simulink model "Therac_Mcode"  (Simulink 8.7)
settings: Solver=FixedStepDiscrete  StartTime=0.0  StopTime=10.0  FixedStep=1  RelTol=1e-3
undefined symbols (not defined in the file or in its folder): sldvsubsys
libraries: simulink x7, sldvlib x2
settings DebuggingCC: SolverPrmCheckMsg=warning  AllowSymbolicDim=off
settings ConfigComp: DVMaxProcessTime=3000  DVMaxTestCaseSteps=500  DVTestSuiteOptimization=CombinedObjectives (Nonlinear Extended)  DVDetectActiveLogic=on

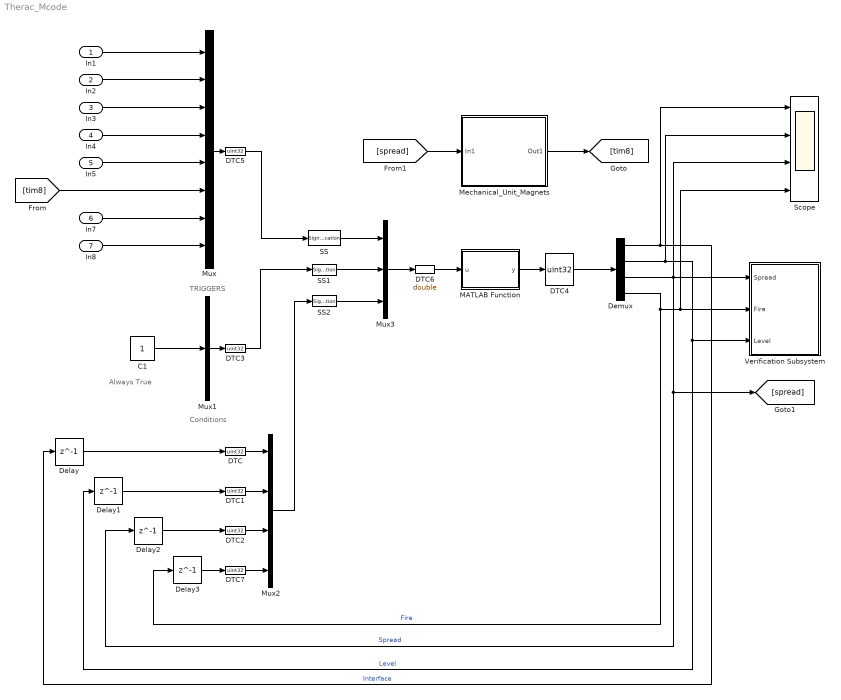
== system Therac_Mcode ==
  note: Always True
  note: Conditions
  note: TRIGGERS
  In1 : Inport  OutDataTypeStr=boolean
  In2 : Inport  Port=2  OutDataTypeStr=boolean
  In3 : Inport  Port=3  OutDataTypeStr=boolean
  In4 : Inport  Port=4  OutDataTypeStr=boolean
  In5 : Inport  Port=5  OutDataTypeStr=boolean
  In7 : Inport  Port=6  OutDataTypeStr=boolean
  In8 : Inport  Port=7  OutDataTypeStr=boolean
  C1 : Constant
  DTC{,1..5,7} (7 alike) : DataTypeConversion  OutDataTypeStr=uint32
  DTC6 : DataTypeConversion  OutDataTypeStr=double
  Delay{,1..3} (4 alike) : Delay  DelayLength=1  InitialCondition=1
  Demux : Demux
  MATLAB Function : MATLAB Function  TreatAsAtomicUnit=on
  Mechanical_Unit_Magnets : Subsystem
  Mux : Mux  Inputs=8
  Mux1 : Mux  Inputs=1
  Mux2 : Mux
  Mux3 : Mux  Inputs=3
  SS : SignalSpecification  Dimensions=8
  SS1 : SignalSpecification  Dimensions=1
  SS2 : SignalSpecification  Dimensions=4
  Scope : Scope  NumInputPorts=4
  Verification Subsystem : Subsystem  Tag=VerificationSubsystem  DisableCoverage=on  LoadFcn=sldvsubsys('check')  TreatAsAtomicUnit=on  SimViewingDevice=on  mask(VerificationSubsystem){}
      mask init:
      | sldvsubsys('maskInit');
      settings: CopyFcn=sldvsubsys('copy');  OpenFcn=open_system(gcb,'force');
      settings: PreSaveFcn=|
      | set_param(gcb,'SimViewingDevice','on');
      | sldvsubsys('check');
      mask Help: helpview(fullfile(docroot,'toolbox','sldv','sldv.map'),'verificationsubsystem')
      mask Display: image(imread('sldvicon_versubsys.png','BackGroundColor',[1 1 1]),'center');
  wires:
  Demux/2 -> Scope/2, Verification Subsystem/3(Level), Delay1/1  "Level"
  Delay2/1 -> DTC2/1
  Mux1/1 -> DTC3/1
  Delay1/1 -> DTC1/1
  Mux/1 -> DTC5/1
  Delay/1 -> DTC/1
  Mux3/1 -> DTC6/1
  Mux2/1 -> SS2/1
  Demux/1 -> Scope/1, Delay/1  "Interface"
  In7/1 -> Mux/7
  In3/1 -> Mux/3
  In2/1 -> Mux/2
  In4/1 -> Mux/4
  In5/1 -> Mux/5
  [tim8] -> Mux/6
  In8/1 -> Mux/8
  MATLAB Function/1(y) -> DTC4/1
  Demux/3 -> Scope/3, Delay2/1, [spread], Verification Subsystem/1(Spread)  "Spread"
  SS/1 -> Mux3/1
  SS1/1 -> Mux3/2
  DTC4/1 -> Demux/1
  DTC/1 -> Mux2/1
  DTC1/1 -> Mux2/2
  DTC2/1 -> Mux2/3
  DTC3/1 -> SS1/1
  SS2/1 -> Mux3/3
  DTC5/1 -> SS/1
  DTC6/1 -> MATLAB Function/1(u)
  In1/1 -> Mux/1
  Delay3/1 -> DTC7/1
  DTC7/1 -> Mux2/4
  Demux/4 -> Delay3/1, Scope/4, Verification Subsystem/2(Fire)  "Fire"
  C1/1 -> Mux1/1
  Mechanical_Unit_Magnets/1(Out1) -> [tim8]
  [spread] -> Mechanical_Unit_Magnets/1(In1)

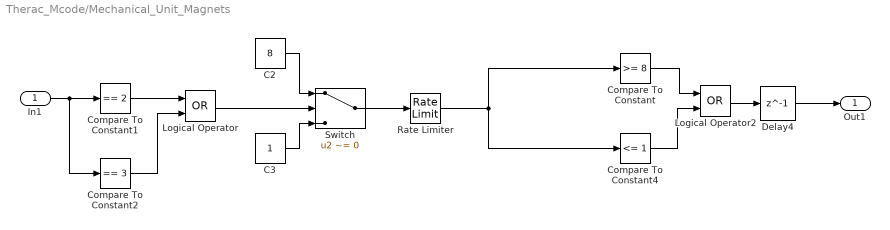
== system Therac_Mcode/Mechanical_Unit_Magnets ==
  In1 : Inport
  C2 : Constant  Value=8
  C3 : Constant
  Compare To Constant : simulink/Logic and Bit Operations/Compare To Constant  relop=>=  const=8  OutDataTypeStr=boolean
  Compare To Constant1 : simulink/Logic and Bit Operations/Compare To Constant  relop===  const=2  OutDataTypeStr=boolean
  Compare To Constant2 : simulink/Logic and Bit Operations/Compare To Constant  relop===  const=3  OutDataTypeStr=boolean
  Compare To Constant4 : simulink/Logic and Bit Operations/Compare To Constant  relop=<=  const=1  OutDataTypeStr=boolean
  Delay4 : Delay  DelayLength=1  InitialCondition=0
  Logical Operator : Logic  Operator=OR  AllPortsSameDT=off  OutDataTypeStr=boolean
  Logical Operator2 : Logic  Operator=OR  AllPortsSameDT=off  OutDataTypeStr=boolean
  Rate Limiter : RateLimiter  SampleTimeMode=inherited
  Switch : Switch  Criteria=u2 ~= 0
  Out1 : Outport
  wires:
  Switch/1 -> Rate Limiter/1
  C3/1 -> Switch/3
  Compare To Constant/1 -> Logical Operator2/1
  Logical Operator/1 -> Switch/2
  Logical Operator2/1 -> Delay4/1
  Compare To Constant4/1 -> Logical Operator2/2
  C2/1 -> Switch/1
  In1/1 -> Compare To Constant2/1, Compare To Constant1/1
  Compare To Constant2/1 -> Logical Operator/2
  Compare To Constant1/1 -> Logical Operator/1
  Rate Limiter/1 -> Compare To Constant/1, Compare To Constant4/1
  Delay4/1 -> Out1/1

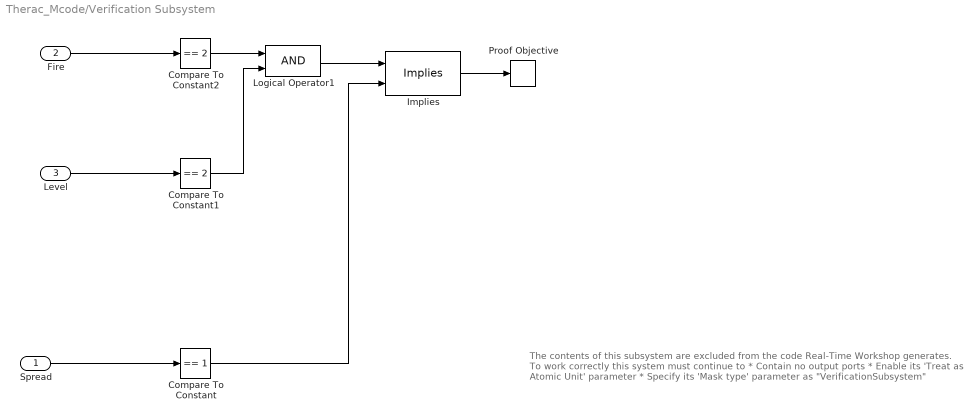
== system Therac_Mcode/Verification Subsystem ==
  note: The contents of this subsystem are excluded from the code Real-Time
      | Workshop generates.
      |
      | To work correctly this system must continue to
      | * Contain no output ports
      | * Enable its 'Treat as Atomic Unit' parameter
      | * Specify its 'Mask type' parameter as "VerificationSubsystem"
  Spread : Inport
  Fire : Inport  Port=2
  Level : Inport  Port=3
  Compare To Constant : simulink/Logic and Bit Operations/Compare To Constant  relop===  const=1  OutDataTypeStr=boolean
  Compare To Constant1 : simulink/Logic and Bit Operations/Compare To Constant  relop===  const=2  OutDataTypeStr=boolean
  Compare To Constant2 : simulink/Logic and Bit Operations/Compare To Constant  relop===  const=2  OutDataTypeStr=boolean
  Implies : sldvlib/Verification Utilities/Implies
  Logical Operator1 : Logic  AllPortsSameDT=off  OutDataTypeStr=boolean
  Proof Objective : sldvlib/Objectives and Constraints/Proof Objective  enabled=on  customAVTBlockType=Proof Objective  intervals=true  dispValues=on  outEnabled=on  enableStopSim=off
      settings: AttributesFormatString=%<intervals>
  wires:
  Implies/1 -> Proof Objective/1
  Spread/1 -> Compare To Constant/1
  Level/1 -> Compare To Constant1/1
  Fire/1 -> Compare To Constant2/1
  Compare To Constant2/1 -> Logical Operator1/1
  Logical Operator1/1 -> Implies/1
  Compare To Constant1/1 -> Logical Operator1/2
  Compare To Constant/1 -> Implies/2

== matlab function MATLAB Function ==
  data: u input double; y output double
function y = fcn(u)
%#codegen
nt = 8 ; nc = 1 ;
Tr = zeros(nt,1); C = zeros(nc,1);
for i = 1:nt; Tr(i) = u(i,1); end  % Assign triggers from input U
for i = 1:nc; C(i) = u(i+nt,1); end % Assign conditions from input U
INTER = u(10,1);
LEVEL = u(11,1);
SPREAD = u(12,1);
FIRE = u(13,1);
% Assign the trigger to one based on priority
% Add additonal conditions to enable triggers here
TRIG = 0;
if  Tr(1) == 1, TRIG = 1;  % UP
elseif  Tr(2) == 1, TRIG = 2;  % ENT
elseif  Tr(3) == 1, TRIG = 3;  % XT
elseif  Tr(4) == 1, TRIG = 4;  % ET
elseif  Tr(5) == 1, TRIG = 5;  % BT
elseif  Tr(6) == 1, TRIG = 6;  % TIM8
elseif  Tr(7) == 1, TRIG = 7;  % RESET
elseif  Tr(8) == 1, TRIG = 8;  % TICK
end
if FIRE == 2
    TRIG = 7;
end

% 1) If in State EDIT AND Trigger XT occurs THEN transit to XBDATAE if condition C1 is True
if  (INTER == 1) && (TRIG == 3) && (C(1) == 1) ; INTER = 4;
% 2) If in State EDIT AND Trigger ET occurs THEN transit to EBDATAE if condition C1 is True
elseif  (INTER == 1) && (TRIG == 4) && (C(1) == 1) ; INTER = 2;
% 3) If in State EBDATAE AND Trigger UP occurs THEN transit to EDIT if condition C1 is True
elseif  (INTER == 2) && (TRIG == 1) && (C(1) == 1) ; INTER = 1;
% 4) If in State EBDATAE AND Trigger ENT occurs THEN transit to EBDATAD if condition C1 is True
elseif  (INTER == 2) && (TRIG == 2) && (C(1) == 1) ; INTER = 3;
% 5) If in State EBDATAD AND Trigger UP occurs THEN transit to EBDATAE if condition C1 is True
elseif  (INTER == 3) && (TRIG == 1) && (C(1) == 1) ; INTER = 2;
% 6) If in State EBDATAD AND Trigger BT occurs THEN transit to TADMIN if condition C1 is True
elseif  (INTER == 3) && (TRIG == 5) && (C(1) == 1) ; INTER = 6;
% 7) If in State XBDATAE AND Trigger UP occurs THEN transit to EDIT if condition C1 is True
elseif  (INTER == 4) && (TRIG == 1) && (C(1) == 1) ; INTER = 1;
% 8) If in State XBDATAE AND Trigger ENT occurs THEN transit to XBDATAD if condition C1 is True
elseif  (INTER == 4) && (TRIG == 2) && (C(1) == 1) ; INTER = 5;
% 9) If in State XBDATAD AND Trigger UP occurs THEN transit to XBDATAE if condition C1 is True
elseif  (INTER == 5) && (TRIG == 1) && (C(1) == 1) ; INTER = 4;
% 10) If in State XBDATAD AND Trigger BT occurs THEN transit to TADMIN if condition C1 is True
elseif  (INTER == 5) && (TRIG == 5) && (C(1) == 1) ; INTER = 6;
% 11) If in State TADMIN AND Trigger ENT occurs THEN transit to EDIT if condition C1 is True
elseif  (INTER == 6) && (TRIG == 2) && (C(1) == 1) ; INTER = 1;
end     
%   ================================================
  
% 12) If in State NEITHER AND Trigger XT occurs THEN transit to XB if condition C1 is True
if  (LEVEL == 1) && (TRIG == 3) && (C(1) == 1) ; LEVEL = 2;
% 13) If in State NEITHER AND Trigger ET occurs THEN transit to EB if condition C1 is True
elseif  (LEVEL == 1) && (TRIG == 4) && (C(1) == 1) ; LEVEL = 3;
% 14) If in State XB AND Trigger ET occurs THEN transit to X2E if condition C1 is True
elseif  (LEVEL == 2) && (TRIG == 4) && (C(1) == 1) ; LEVEL = 4;
% 15) If in State XB AND Trigger RESET occurs THEN transit to NEITHER if condition C1 is True
elseif  (LEVEL == 2) && (TRIG == 7) && (C(1) == 1) ; LEVEL = 1;
% 16) If in State EB AND Trigger XT occurs THEN transit to E2X if condition C1 is True
elseif  (LEVEL == 3) && (TRIG == 3) && (C(1) == 1) ; LEVEL = 5;
% 17) If in State EB AND Trigger RESET occurs THEN transit to NEITHER if condition C1 is True
elseif  (LEVEL == 3) && (TRIG == 7) && (C(1) == 1) ; LEVEL = 1;
% 18) If in State X2E AND Trigger TICK occurs THEN transit to EB if condition C1 is True
elseif  (LEVEL == 4) && (TRIG == 8) && (C(1) == 1) ; LEVEL = 3;
% 19) If in State E2X AND Trigger TICK occurs THEN transit to XB if condition C1 is True
elseif  (LEVEL == 5) && (TRIG == 8) && (C(1) == 1) ; LEVEL = 2;
end     
%   ================================================
  
% 20) If in State INPLACE AND Trigger ET occurs THEN transit to MOVOUT if condition C1 is True
if  (SPREAD == 1) && (TRIG == 4) && (C(1) == 1) ; SPREAD = 2;
% 21) If in State MOVOUT AND Trigger XT occurs THEN transit to MOVIN if condition C1 is True
elseif  (SPREAD == 2) && (TRIG == 3) && (C(1) == 1) ; SPREAD = 4;
% 22) If in State MOVOUT AND Trigger TIM8 occurs THEN transit to OUTPLACE if condition C1 is True
elseif  (SPREAD == 2) && (TRIG == 6) && (C(1) == 1) ; SPREAD = 3;
% 23) If in State OUTPLACE AND Trigger XT occurs THEN transit to MOVIN if condition C1 is True
elseif  (SPREAD == 3) && (TRIG == 3) && (C(1) == 1) ; SPREAD = 4;
% 24) If in State MOVIN AND Trigger ET occurs THEN transit to MOVOUT if condition C1 is True
elseif  (SPREAD == 4) && (TRIG == 4) && (C(1) == 1) ; SPREAD = 2;
% 25) If in State MOVIN AND Trigger TIM8 occurs THEN transit to INPLACE if condition C1 is True
elseif  (SPREAD == 4) && (TRIG == 6) && (C(1) == 1) ; SPREAD = 1;
end     
%   ================================================
  
% 26) If in State WAIT AND Trigger BT occurs THEN transit to FIRED if condition C1 is True
if  (FIRE == 1) && (TRIG == 5) && (C(1) == 1) ; FIRE = 2;
% 27) If in State FIRED AND Trigger TICK occurs THEN transit to WAIT if condition C1 is True
elseif  (FIRE == 2) && (TRIG == 8) && (C(1) == 1) ; FIRE = 1;
end     
%   ================================================
  
% ============== Set the outputs ===========
y = zeros(4,1);
y(1) = INTER;
y(2) = LEVEL;
y(3) = SPREAD;
y(4) = FIRE;
